simulink model "lab_4_simulink"  (R2024a)
settings: Solver=ode4  StartTime=0.0  StopTime=10.0  FixedStep=1/128  MaxStep=1/128  RelTol=1e-3
libraries: simulink x1
settings Model: Creator=lw53894  LastModifiedBy=lw53894

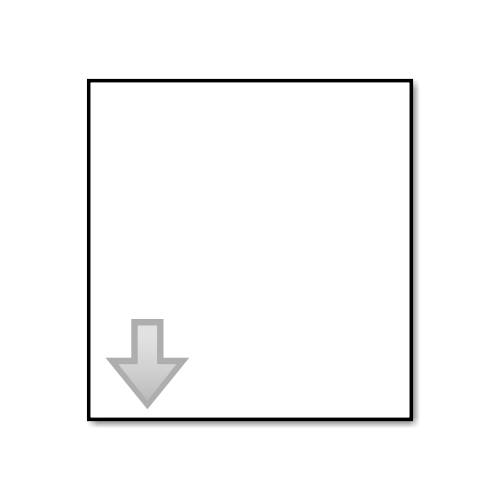
[thumbnail: Simulink's stored preview of the top-level diagram]
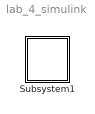
== system lab_4_simulink ==
  Subsystem1 : Subsystem  mask{M=250, R=5, G=9.81, rs=0.2, Vx=10, Vy=5, x=2, y=7}

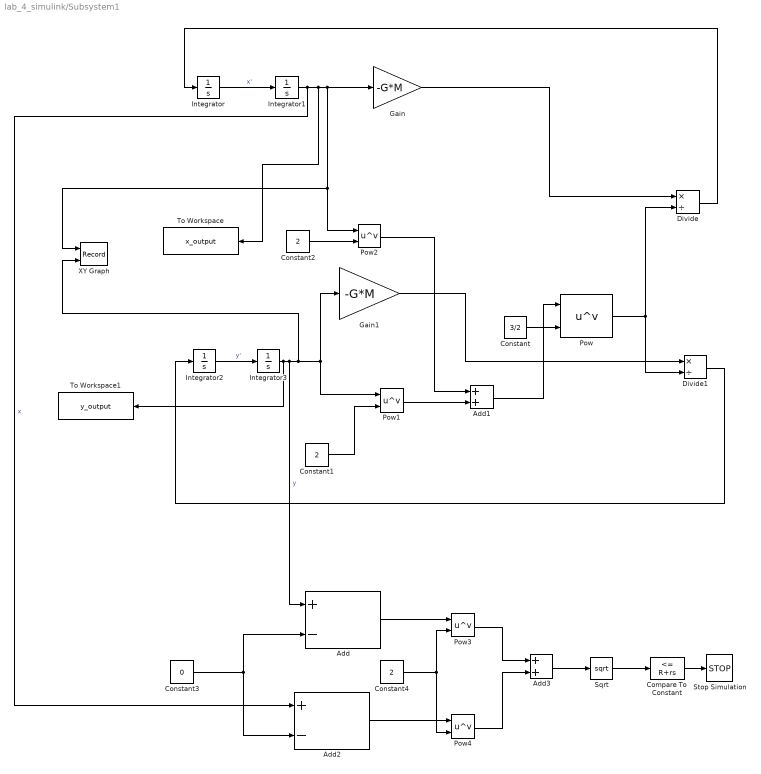
== system lab_4_simulink/Subsystem1 ==
  Add : Sum  Inputs=+-
  Add1 : Sum
  Add2 : Sum  Inputs=+-
  Add3 : Sum
  Compare To Constant : simulink/Logic and Bit Operations/Compare To Constant  relop=<=  const=R+rs  OutDataTypeStr=boolean
  Constant : Constant  Value=3/2
  Constant1 : Constant  Value=2
  Constant2 : Constant  Value=2
  Constant3 : Constant  Value=0
  Constant4 : Constant  Value=2
  Divide : Product  Inputs=*/
  Divide1 : Product  Inputs=*/
  Gain : Gain  Gain=-G*M
  Gain1 : Gain  Gain=-G*M
  Integrator : Integrator  InitialCondition=Vx
  Integrator1 : Integrator  InitialCondition=x
  Integrator2 : Integrator  InitialCondition=Vy
  Integrator3 : Integrator  InitialCondition=y
  Pow{,1..4} (5 alike) : Math  Operator=pow  RndMeth=Zero
  Sqrt : Sqrt
  Stop Simulation : Stop
  To Workspace : ToWorkspace  VariableName=x_output  SaveFormat=Timeseries  SampleTime=-1
  To Workspace1 : ToWorkspace  VariableName=y_output  SaveFormat=Timeseries  SampleTime=-1
  XY Graph : Record  FileSettingsInternal="{\"entries\":[{\"content\":{\"excelSettings\":{\"content\":{},\"type\":\"Streamout.ExcelSettings\"}},\"type\":\"Streamout.FileSettingStorage\",\"uuid\":\"\"}],\"packageUris\":[\"http:\\/\\/schema.mathworks.com\\/mf0\\/streamout_blocks\\/R2020a\"],\"version\":\"1.0\"}"  Layout=[1 1]  SignalsInternal="{\"entries\":[{\"content\":{\"signals\":[{\"content\":{\"blockPath\":[],\"dimensions\":[1],\"domain\":\"\",\"lineColor\":\"#a2142f\",\"plots\":[ 1 ],\"port\":1,\"sid\":[\"\"],\"signalID\":1,\"signalName\":\"x\"},\"type\":\"RecordBlkView.Signal\",\"uuid\":\"\"},{\"content\":{\"blockPath\":[],\"dimensions\":[1],\"domain\":\"\",\"lineColor\":\"#139fff\",\"plots\":[ 1 ],\"port\":2,\"sid\":[\"\"],\"signalID\":2,\"signalName\":\"y\"},\"type\":\"RecordBlkView.Signal\",\"uuid\":\"\"}]},\"type\":\"RecordBlkView.InputSignals\",\"uuid\":\"\"}],\"packageUris\":[\"http:\\/\\/schema.mathworks.com\\/mf0\\/streamout_blocks\\/R2020a\"],\"version\":\"1.0\"}"  VisualizationBindings="{\"xyplotplugin\":{\"info\":[{\"series\":[{\"bindingParametersList\":[{\"parameter\":\"X-Axis\",\"signalID\":1,\"signalName\":\"x\"},{\"parameter\":\"Y-Axis\",\"signalID\":2,\"signalName\":\"y\"}],\"seriesID\":0}],\"subplotID\":1}]}}"  CompatibilityTag=XY
  wires:
  Add1/1 -> Pow/1
  Gain1/1 -> Divide1/1
  Integrator3/1 -> To Workspace1/1, Add/1, XY Graph/2, Pow1/1, Gain1/1  "y"
  Integrator/1 -> Integrator1/1  "x'"
  Pow/1 -> Divide1/2, Divide/2
  Integrator1/1 -> Add2/1, To Workspace/1, Pow2/1, XY Graph/1, Gain/1  "x"
  Integrator2/1 -> Integrator3/1  "y'"
  Pow1/1 -> Add1/2
  Constant1/1 -> Pow1/2
  Gain/1 -> Divide/1
  Pow2/1 -> Add1/1
  Constant2/1 -> Pow2/2
  Divide/1 -> Integrator/1
  Divide1/1 -> Integrator2/1
  Constant/1 -> Pow/2
  Constant3/1 -> Add/2, Add2/2
  Constant4/1 -> Pow3/2, Pow4/2
  Add/1 -> Pow3/1
  Add2/1 -> Pow4/1
  Pow3/1 -> Add3/1
  Pow4/1 -> Add3/2
  Add3/1 -> Sqrt/1
  Sqrt/1 -> Compare To Constant/1
  Compare To Constant/1 -> Stop Simulation/1
